simulink model "deployAGV_stateflow"  (R2024a)
settings: configuration reference "SharedConfig" (kept outside this file)
PostLoadFcn:
  | AGV_simulation
model workspace (MAT data in the model file):
  L = Simulink.Parameter
  L.Value = 2
  L.Complexity = 'real'
  L.Dimensions = [1 1]
  L.DataType = 'auto'
  mdlWSDbList = ["C:\Users\matlab.cut\Desktop\AMR\canbus_files\tramontina_database_xsens.dbc" "tramontina_database_curtis.dbc"]
  mdlWSDbcList = ["C:\Users\rodri\Dev\Projects\External\Tramontina\atlas\interface_models\xsens.dbc" "tramontina_database_curtis.dbc"]
  tfinal = Simulink.Parameter
  tfinal.Value = 350
  tfinal.Complexity = 'real'
  tfinal.Dimensions = [1 1]
  tfinal.DataType = 'auto'
undefined symbols (not defined in the file): DiscIntNeverNeededParam, magnitude, num_of_wps, T, T5, tstep
libraries: simulink x1, slrealtimeloglib x1
settings Model: DataDictionary=configuration_dictionary.sldd  Creator=rodri  LastModifiedBy=matlab.cut
settings ConfigSetRef: SourceName=SharedConfig

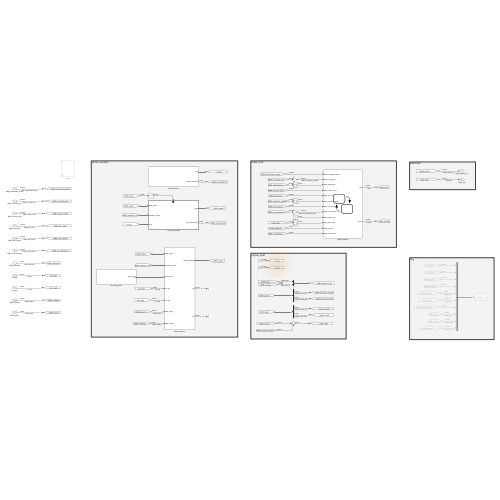
[thumbnail: Simulink's stored preview of the top-level diagram]
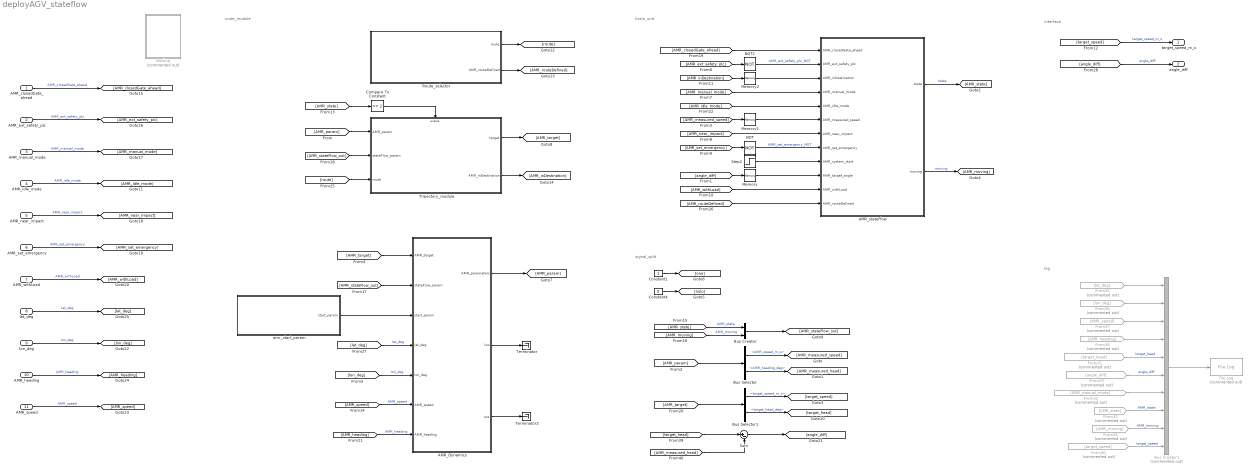
== system deployAGV_stateflow ==
  note: route_module
  note: brain_unit
  note: signal_split
  note: interface
  note: log
  AMR_closedGate_ahead : Inport  OutDataTypeStr=boolean
  AMR_ext_safety_plc : Inport  Port=2  OutDataTypeStr=boolean
  AMR_manual_mode : Inport  Port=3  OutDataTypeStr=boolean
  AMR_idle_mode : Inport  Port=4  OutDataTypeStr=boolean
  AMR_near_impact : Inport  Port=5  OutDataTypeStr=boolean
  AMR_set_emergency : Inport  Port=6  OutDataTypeStr=boolean
  AMR_withLoad : Inport  Port=7
  lat_deg : Inport  Port=8
  lon_deg : Inport  Port=9
  AMR_heading : Inport  Port=10
  AMR_speed : Inport  Port=11
  AMR_Dynamics : Subsystem
  AMR_stateFlow : Stateflow chart  TreatAsAtomicUnit=on
  Backup : Subsystem  Commented=on
  Bus Creator : BusCreator  Inputs=2
  Bus Creator1 : BusCreator  Commented=on  Inputs=10
  Bus Selector : BusSelector  OutputSignals=AMR_speed_m_s,AMR_heading_deg
  Bus Selector1 : BusSelector  OutputSignals=target_speed_m_s,target_head_deg
  Compare To Constant : simulink/Logic and Bit Operations/Compare To Constant  relop===  const=2  OutDataTypeStr=boolean
  Constant1 : Constant
  Constant4 : Constant  Value=0
  File Log : slrealtimeloglib/File Log  Commented=on  decimation=1  inputProcessing=Elements as channels (sample based)
  From29 : From  Commented=on  GotoTag=angle_diff
  From30 : From  Commented=on  GotoTag=target_speed
  From31 : From  Commented=on  GotoTag=target_head
  From32 : From  Commented=on  GotoTag=AMR_manual_mode
  From33 : From  Commented=on  GotoTag=AMR_state
  From34 : From  Commented=on  GotoTag=AMR_moving
  From35 : From  Commented=on  GotoTag=lat_deg
  From36 : From  Commented=on  GotoTag=lon_deg
  From37 : From  Commented=on  GotoTag=AMR_speed
  From38 : From  Commented=on  GotoTag=AMR_heading
  Memory : Memory
  Memory1 : Memory
  Memory2 : Memory
  NOT : Logic  Operator=NOT  IconShape=distinctive  AllPortsSameDT=off  OutDataTypeStr=boolean
  NOT1 : Logic  Operator=NOT  IconShape=distinctive  AllPortsSameDT=off  OutDataTypeStr=boolean
  Route_selector : Subsystem
  Step2 : Step  Time=10  SampleTime=0
  Sum : Sum  Inputs=|+-
  Terminator : Terminator
  Terminator2 : Terminator
  Trajectory_module : Subsystem
  amr_start_param : Subsystem
  target_speed_m_s : Outport
  angle_diff : Outport  Port=2
  wires:
  AMR_stateFlow/2(moving) -> [AMR_moving]  "moving"
  AMR_stateFlow/1(state) -> [AMR_state]  "state"
  [AMR_ext_safety_plc] -> NOT1/1
  [AMR_manual_mode] -> AMR_stateFlow/4(AMR_manual_mode)
  [AMR_measured_speed] -> Memory1/1
  [AMR_near_impact] -> AMR_stateFlow/7(AMR_near_impact)
  [AMR_set_emergency] -> NOT/1
  Step2/1 -> AMR_stateFlow/9(AMR_system_start)
  [angle_diff] -> Memory/1
  [AMR_withLoad] -> AMR_stateFlow/11(AMR_withLoad)
  [AMR_inDestination] -> Memory2/1
  [AMR_closedGate_ahead] -> AMR_stateFlow/1(AMR_closedGate_ahead)
  AMR_Dynamics/1(AMR_parameters) -> [AMR_param]
  [AMR_param] -> Trajectory_module/1(AMR_param)
  Trajectory_module/1(target) -> [AMR_target]
  [AMR_target] -> AMR_Dynamics/1(AMR_target)
  amr_start_param/1(start_param) -> AMR_Dynamics/3(start_param)
  [AMR_stateFlow_out] -> AMR_Dynamics/2(stateFlow_param)
  [AMR_stateFlow_out] -> Trajectory_module/2(stateFlow_param)
  [AMR_state] -> Compare To Constant/1
  Compare To Constant/1 -> Trajectory_module/Enable
  Memory/1 -> AMR_stateFlow/10(AMR_target_angle)
  Memory1/1 -> AMR_stateFlow/6(AMR_measured_speed)
  Route_selector/1(route) -> [route]
  Route_selector/2(AMR_routeDefined) -> [AMR_routeDefined]
  [route] -> Trajectory_module/3(route)
  [AMR_routeDefined] -> AMR_stateFlow/12(AMR_routeDefined)
  Trajectory_module/2(AMR_inDestination) -> [AMR_inDestination]
  Memory2/1 -> AMR_stateFlow/3(AMR_inDestination)
  AMR_closedGate_ahead/1 -> [AMR_closedGate_ahead]  "AMR_closedGate_ahead"
  AMR_manual_mode/1 -> [AMR_manual_mode]  "AMR_manual_mode"
  AMR_near_impact/1 -> [AMR_near_impact]  "AMR_near_impact"
  AMR_withLoad/1 -> [AMR_withLoad]  "AMR_withLoad"
  lat_deg/1 -> [lat_deg]  "lat_deg"
  [lat_deg] -> AMR_Dynamics/4(lat_deg)  "lat_deg"
  lon_deg/1 -> [lon_deg]  "lon_deg"
  AMR_speed/1 -> [AMR_speed]  "AMR_speed"
  AMR_heading/1 -> [AMR_heading]  "AMR_heading"
  [lon_deg] -> AMR_Dynamics/5(lon_deg)  "lon_deg"
  [AMR_speed] -> AMR_Dynamics/6(AMR_speed)  "AMR_speed"
  [AMR_heading] -> AMR_Dynamics/7(AMR_heading)  "AMR_heading"
  AMR_Dynamics/3(rws) -> Terminator2/1
  AMR_Dynamics/2(lws) -> Terminator/1
  AMR_set_emergency/1 -> [AMR_set_emergency]  "AMR_set_emergency"
  AMR_ext_safety_plc/1 -> [AMR_ext_safety_plc]  "AMR_ext_safety_plc"
  NOT1/1 -> AMR_stateFlow/2(AMR_ext_safety_plc)  "AMR_ext_safety_plc_NOT"
  NOT/1 -> AMR_stateFlow/8(AMR_set_emergency)  "AMR_set_emergency_NOT"
  Bus Creator/1 -> [AMR_stateFlow_out]
  [AMR_moving] -> Bus Creator/2  "AMR_moving"
  [AMR_state] -> Bus Creator/1  "AMR_state"
  Bus Selector/1 -> [AMR_measured_speed]  "<AMR_speed_m_s>"
  Bus Selector1/2 -> [target_head]  "<target_head_deg>"
  Constant1/1 -> [one]
  Constant4/1 -> [nulo]
  Bus Selector/2 -> [AMR_measured_head]  "<AMR_heading_deg>"
  Bus Selector1/1 -> [target_speed]  "<target_speed_m_s>"
  [AMR_param] -> Bus Selector/1
  [AMR_target] -> Bus Selector1/1
  [angle_diff] -> angle_diff/1  "angle_diff"
  [target_speed] -> target_speed_m_s/1  "target_speed_m_s"
  From38/1 -> Bus Creator1/4
  From31/1 -> Bus Creator1/5  "target_head"
  From35/1 -> Bus Creator1/1
  From36/1 -> Bus Creator1/2
  From29/1 -> Bus Creator1/6  "angle_diff"
  From34/1 -> Bus Creator1/9  "AMR_moving"
  From30/1 -> Bus Creator1/10  "target_speed"
  Bus Creator1/1 -> File Log/1
  From33/1 -> Bus Creator1/8  "AMR_state"
  From37/1 -> Bus Creator1/3
  From32/1 -> Bus Creator1/7
  [AMR_measured_head] -> Sum/2
  [target_head] -> Sum/1
  Sum/1 -> [angle_diff]
  AMR_idle_mode/1 -> [AMR_idle_mode]  "AMR_idle_mode"
  [AMR_idle_mode] -> AMR_stateFlow/5(AMR_idle_mode)

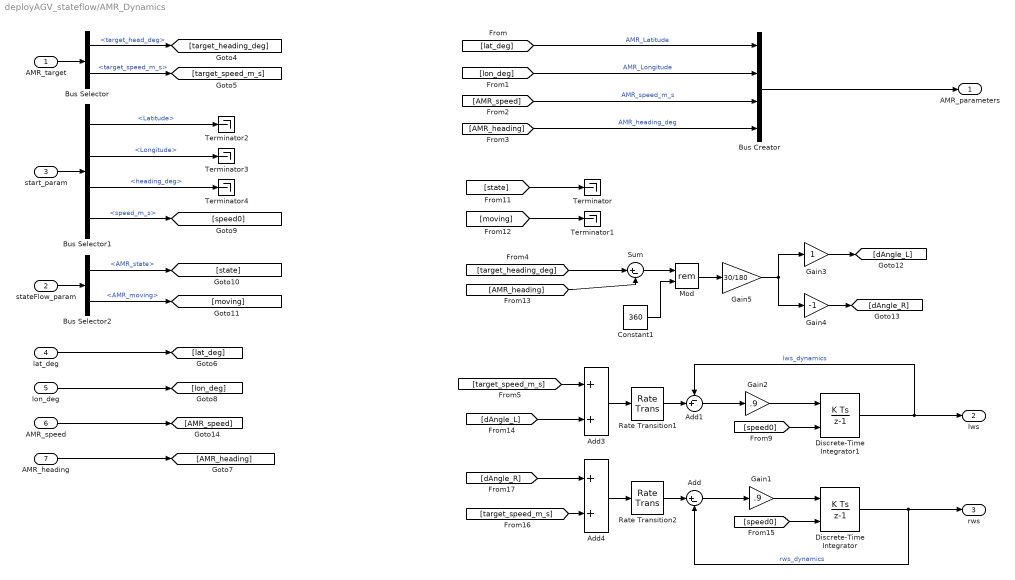
== system deployAGV_stateflow/AMR_Dynamics ==
  AMR_target : Inport
  stateFlow_param : Inport  Port=2
  start_param : Inport  Port=3
  lat_deg : Inport  Port=4
  lon_deg : Inport  Port=5
  AMR_speed : Inport  Port=6
  AMR_heading : Inport  Port=7
  Add : Sum  Inputs=|+-
  Add1 : Sum  Inputs=-+|
  Add3 : Sum
  Add4 : Sum
  Bus Creator : BusCreator  Inputs=4
  Bus Selector : BusSelector  OutputSignals=target_head_deg,target_speed_m_s
  Bus Selector1 : BusSelector  OutputSignals=Latitude,Longitude,heading_deg,speed_m_s
  Bus Selector2 : BusSelector  OutputSignals=AMR_state,AMR_moving
  Constant1 : Constant  Value=360
  Discrete-Time Integrator : DiscreteIntegrator  InitialConditionSource=external  SampleTime=tstep  ICPrevOutput=DiscIntNeverNeededParam  ICPrevScaledInput=DiscIntNeverNeededParam
  Discrete-Time Integrator1 : DiscreteIntegrator  InitialConditionSource=external  SampleTime=tstep  ICPrevOutput=DiscIntNeverNeededParam  ICPrevScaledInput=DiscIntNeverNeededParam
  Gain1 : Gain  Gain=.9
  Gain2 : Gain  Gain=.9
  Gain3 : Gain
  Gain4 : Gain  Gain=-1
  Gain5 : Gain  Gain=30/180
  Mod : Math  Operator=rem
  Rate Transition1 : RateTransition
  Rate Transition2 : RateTransition
  Sum : Sum  Inputs=|+-
  Terminator{,1..4} (5 alike) : Terminator
  AMR_parameters : Outport
  lws : Outport  Port=2
  rws : Outport  Port=3
  wires:
  [lat_deg] -> Bus Creator/1  "AMR_Latitude"
  [lon_deg] -> Bus Creator/2  "AMR_Longitude"
  Bus Creator/1 -> AMR_parameters/1
  [AMR_speed] -> Bus Creator/3  "AMR_speed_m_s"
  [AMR_heading] -> Bus Creator/4  "AMR_heading_deg"
  AMR_target/1 -> Bus Selector/1
  start_param/1 -> Bus Selector1/1
  Bus Selector/1 -> [target_heading_deg]  "<target_head_deg>"
  Bus Selector/2 -> [target_speed_m_s]  "<target_speed_m_s>"
  Bus Selector1/1 -> Terminator2/1  "<Latitude>"
  Bus Selector1/2 -> Terminator3/1  "<Longitude>"
  Bus Selector1/3 -> Terminator4/1  "<heading_deg>"
  Bus Selector1/4 -> [speed0]  "<speed_m_s>"
  [target_heading_deg] -> Sum/1
  stateFlow_param/1 -> Bus Selector2/1
  Bus Selector2/2 -> [moving]  "<AMR_moving>"
  Bus Selector2/1 -> [state]  "<AMR_state>"
  [state] -> Terminator/1
  [moving] -> Terminator1/1
  [AMR_heading] -> Sum/2
  Discrete-Time Integrator1/1 -> Add1/1, lws/1  "lws_dynamics"
  Discrete-Time Integrator/1 -> Add/2, rws/1  "rws_dynamics"
  [speed0] -> Discrete-Time Integrator/2
  Add/1 -> Gain1/1
  Add1/1 -> Gain2/1
  [speed0] -> Discrete-Time Integrator1/2
  Sum/1 -> Mod/1
  Constant1/1 -> Mod/2
  Gain3/1 -> [dAngle_L]
  Gain2/1 -> Discrete-Time Integrator1/1
  Gain1/1 -> Discrete-Time Integrator/1
  Gain4/1 -> [dAngle_R]
  Add3/1 -> Rate Transition1/1
  [target_speed_m_s] -> Add4/2
  Mod/1 -> Gain5/1
  [dAngle_R] -> Add4/1
  Gain5/1 -> Gain3/1, Gain4/1
  Add4/1 -> Rate Transition2/1
  lat_deg/1 -> [lat_deg]
  lon_deg/1 -> [lon_deg]
  AMR_speed/1 -> [AMR_speed]
  AMR_heading/1 -> [AMR_heading]
  [target_speed_m_s] -> Add3/1
  [dAngle_L] -> Add3/2
  Rate Transition1/1 -> Add1/2
  Rate Transition2/1 -> Add/1

== system deployAGV_stateflow/Backup ==
  Add : Sum  Inputs=+-
  Constant5 : Constant  Value=0
  GPS : Subsystem  Commented=on
  GPS_speed_measure : Subsystem  Commented=on
  Step : Step  Time=10  After=.000005  SampleTime=0
  Step1 : Step  Time=50  After=.000005  SampleTime=0
  wires:
  GPS_speed_measure/2(heading_deg) -> [agv_measured_heading]
  GPS/1(POS) -> [agv_pos]
  Constant5/1 -> GPS/1(dlat)
  Step1/1 -> Add/2
  Add/1 -> GPS/2(dlng)
  [agv_pos] -> GPS_speed_measure/1(GPS_POS)
  Step/1 -> Add/1
  GPS_speed_measure/1(speed_m_s) -> [agv_measured_speed]

== system deployAGV_stateflow/Route_selector ==
  Add : Sum  Inputs=+-
  Bus Creator4 : BusCreator  Inputs=2
  Constant : Constant
  Constant5 : Constant  Value=T.Latitude
  Constant9 : Constant  Value=T.Longitude
  Step : Step  Time=15  SampleTime=0
  Step1 : Step  Time=20  SampleTime=0
  Terminator : Terminator
  route : Outport
  AMR_routeDefined : Outport  Port=2
  wires:
  Bus Creator4/1 -> route/1  "route"
  Step/1 -> Add/1
  Step1/1 -> Add/2
  Constant9/1 -> Bus Creator4/2  "Longitude"
  Constant5/1 -> Bus Creator4/1  "Latitude"
  Constant/1 -> AMR_routeDefined/1
  Add/1 -> Terminator/1

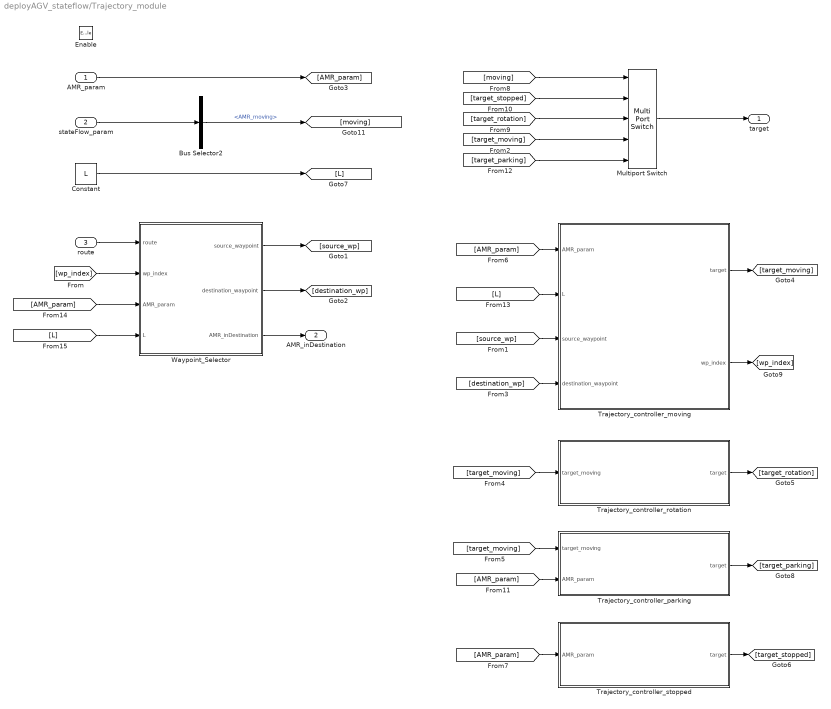
== system deployAGV_stateflow/Trajectory_module ==
  AMR_param : Inport
  stateFlow_param : Inport  Port=2
  route : Inport  Port=3
  Enable : EnablePort
  Bus Selector2 : BusSelector  OutputSignals=AMR_moving
  Constant : Constant  Value=L
  Multiport Switch : MultiPortSwitch  DataPortOrder=Zero-based contiguous  Inputs=4  zeroidx=on  SaturateOnIntegerOverflow=off  InputSameDT=off
  Trajectory_controller_moving : Subsystem
  Trajectory_controller_parking : Subsystem
  Trajectory_controller_rotation : Subsystem
  Trajectory_controller_stopped : Subsystem
  Waypoint_Selector : Subsystem
  target : Outport
  AMR_inDestination : Outport  Port=2
  wires:
  Trajectory_controller_moving/2(wp_index) -> [wp_index]
  [wp_index] -> Waypoint_Selector/2(wp_index)
  Trajectory_controller_moving/1(target) -> [target_moving]
  route/1 -> Waypoint_Selector/1(route)
  [L] -> Trajectory_controller_moving/2(L)
  Bus Selector2/1 -> [moving]  "<AMR_moving>"
  stateFlow_param/1 -> Bus Selector2/1
  [source_wp] -> Trajectory_controller_moving/3(source_waypoint)
  Waypoint_Selector/1(source_waypoint) -> [source_wp]
  Waypoint_Selector/2(destination_waypoint) -> [destination_wp]
  [destination_wp] -> Trajectory_controller_moving/4(destination_waypoint)
  AMR_param/1 -> [AMR_param]
  [AMR_param] -> Trajectory_controller_moving/1(AMR_param)
  Trajectory_controller_rotation/1(target) -> [target_rotation]
  Multiport Switch/1 -> target/1
  [moving] -> Multiport Switch/1
  [target_stopped] -> Multiport Switch/2
  [target_parking] -> Multiport Switch/5
  [target_moving] -> Multiport Switch/4
  [target_rotation] -> Multiport Switch/3
  [target_moving] -> Trajectory_controller_rotation/1(target_moving)
  [target_moving] -> Trajectory_controller_parking/1(target_moving)
  Trajectory_controller_parking/1(target) -> [target_parking]
  [AMR_param] -> Trajectory_controller_parking/2(AMR_param)
  [AMR_param] -> Trajectory_controller_stopped/1(AMR_param)
  Trajectory_controller_stopped/1(target) -> [target_stopped]
  Constant/1 -> [L]
  [AMR_param] -> Waypoint_Selector/3(AMR_param)
  [L] -> Waypoint_Selector/4(L)
  Waypoint_Selector/3(AMR_inDestination) -> AMR_inDestination/1

== system deployAGV_stateflow/amr_start_param ==
  Bus Creator : BusCreator  Inputs=4
  Constant : Constant  Value=T5.Latitude(1)
  Constant1 : Constant  Value=T5.Longitude(1)
  Constant2 : Constant  Value=0
  Constant3 : Constant  Value=0
  start_param : Outport
  wires:
  Bus Creator/1 -> start_param/1
  Constant/1 -> Bus Creator/1  "Latitude"
  Constant1/1 -> Bus Creator/2  "Longitude"
  Constant2/1 -> Bus Creator/3  "heading_deg"
  Constant3/1 -> Bus Creator/4  "speed_m_s"

== system deployAGV_stateflow/Backup/GPS ==
  dlat : Inport
  dlng : Inport  Port=2
  Add : Sum  Inputs=|++
  Add1 : Sum  Inputs=|++
  Matrix Concatenate : Concatenate  Mode=Multidimensional array  ConcatenateDimension=2
  lat : Memory  InitialCondition=-29.272334
  lng : Memory  InitialCondition=-51.467679
  POS : Outport
  wires:
  lat/1 -> Add1/2, Matrix Concatenate/1
  Matrix Concatenate/1 -> POS/1
  dlat/1 -> Add1/1
  Add1/1 -> lat/1
  lng/1 -> Add/2, Matrix Concatenate/2
  Add/1 -> lng/1
  dlng/1 -> Add/1

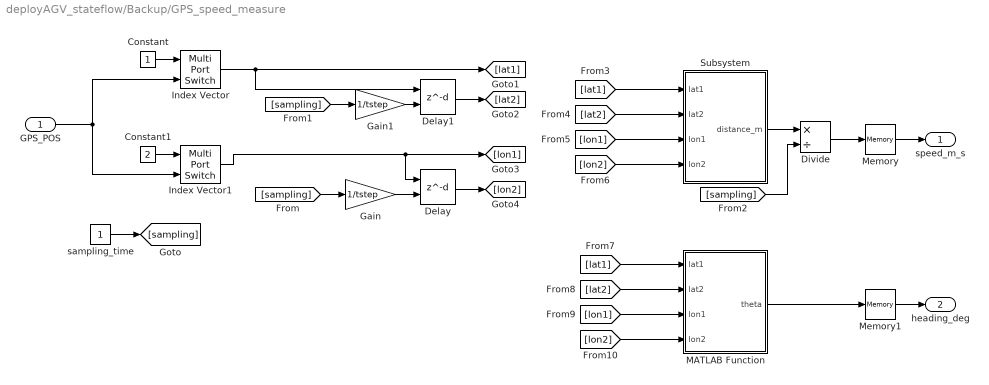
== system deployAGV_stateflow/Backup/GPS_speed_measure ==
  GPS_POS : Inport
  Constant : Constant
  Constant1 : Constant  Value=2
  Delay : Delay  DelayLengthSource=Input port  DelayLength=5/tstep  InitialCondition=-51.467679
      settings: InputPortMap=u0,p1
  Delay1 : Delay  DelayLengthSource=Input port  DelayLength=5/tstep  InitialCondition=-29.272334
      settings: InputPortMap=u0,p1
  Divide : Product  Inputs=*/
  Gain : Gain  Gain=1/tstep
  Gain1 : Gain  Gain=1/tstep
  Index Vector : MultiPortSwitch  Inputs=1  SaturateOnIntegerOverflow=off  InputSameDT=off
  Index Vector1 : MultiPortSwitch  Inputs=1  SaturateOnIntegerOverflow=off  InputSameDT=off
  MATLAB Function : MATLAB Function  TreatAsAtomicUnit=on
  Memory : Memory
  Memory1 : Memory
  Subsystem : Subsystem
  sampling_time : Constant
  speed_m_s : Outport
  heading_deg : Outport  Port=2
  wires:
  Subsystem/1(distance_m) -> Divide/1
  Memory/1 -> speed_m_s/1
  Divide/1 -> Memory/1
  Constant/1 -> Index Vector/1
  Constant1/1 -> Index Vector1/1
  Index Vector1/1 -> [lon1], Delay/1
  sampling_time/1 -> [sampling]
  Gain/1 -> Delay/2
  [sampling] -> Gain/1
  [sampling] -> Gain1/1
  Gain1/1 -> Delay1/2
  Index Vector/1 -> [lat1], Delay1/1
  GPS_POS/1 -> Index Vector/2, Index Vector1/2
  [sampling] -> Divide/2
  Memory1/1 -> heading_deg/1
  Delay1/1 -> [lat2]
  Delay/1 -> [lon2]
  [lat2] -> Subsystem/2(lat2)
  [lon1] -> Subsystem/3(lon1)
  [lon2] -> Subsystem/4(lon2)
  [lat1] -> Subsystem/1(lat1)
  [lon2] -> MATLAB Function/4(lon2)
  [lat1] -> MATLAB Function/1(lat1)
  [lon1] -> MATLAB Function/3(lon1)
  [lat2] -> MATLAB Function/2(lat2)
  MATLAB Function/1(theta) -> Memory1/1

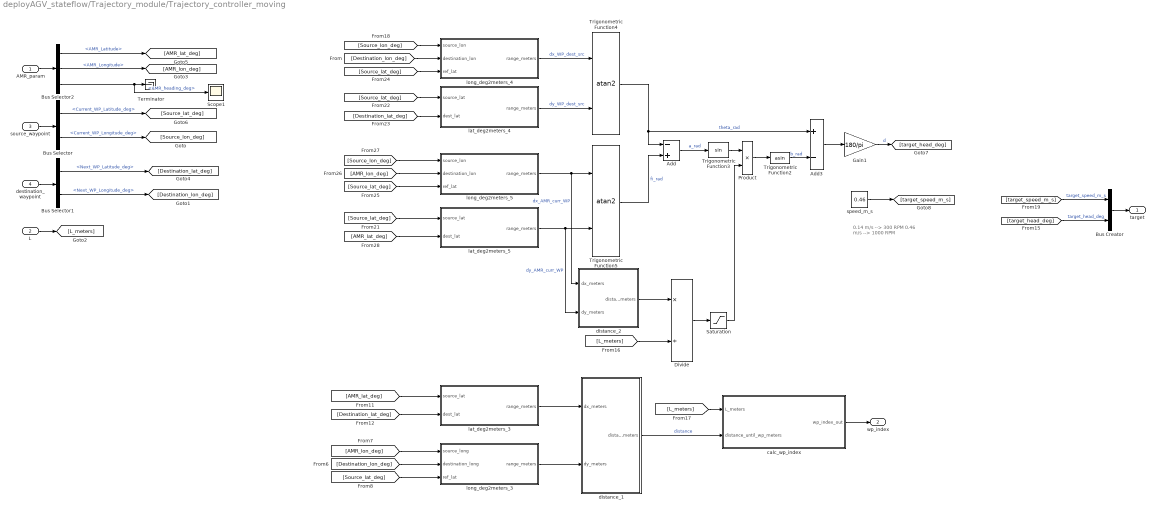
== system deployAGV_stateflow/Trajectory_module/Trajectory_controller_moving ==
  note: 0.14 m/s --> 300 RPM
      | 0.46 m/s --> 1000 RPM
  AMR_param : Inport
  L : Inport  Port=2
  source_waypoint : Inport  Port=3
  destination_waypoint : Inport  Port=4
  Add : Sum  Inputs=-+
  Add3 : Sum  Inputs=+-
  Bus Creator : BusCreator  Inputs=2
  Bus Selector : BusSelector  OutputSignals=Current_WP_Latitude_deg,Current_WP_Longitude_deg
  Bus Selector1 : BusSelector  OutputSignals=Next_WP_Latitude_deg,Next_WP_Longitude_deg
  Bus Selector2 : BusSelector  OutputSignals=AMR_Latitude,AMR_Longitude,AMR_heading_deg
  Divide : Product  Inputs=*/
  Gain1 : Gain  Gain=180/pi
  Product : Product
  Saturation : Saturate  UpperLimit=1  LowerLimit=0
  Scope1 : Scope
  Terminator : Terminator
  Trigonometric Function2 : Trigonometry  Operator=asin
  Trigonometric Function3 : Trigonometry
  Trigonometric Function4 : Trigonometry  Operator=atan2
  Trigonometric Function5 : Trigonometry  Operator=atan2
  calc_wp_index : Subsystem
  distance_1 : Subsystem  TreatAsAtomicUnit=on
  distance_2 : Subsystem  TreatAsAtomicUnit=on
  lat_deg2meters_3 : Subsystem  TreatAsAtomicUnit=on
  lat_deg2meters_4 : Subsystem  TreatAsAtomicUnit=on
  lat_deg2meters_5 : Subsystem  TreatAsAtomicUnit=on
  long_deg2meters_3 : Subsystem  TreatAsAtomicUnit=on
  long_deg2meters_4 : Subsystem  TreatAsAtomicUnit=on
  long_deg2meters_5 : Subsystem  TreatAsAtomicUnit=on
  speed_m_s : Constant  Value=0.46
  target : Outport
  wp_index : Outport  Port=2
  wires:
  distance_1/1(distance_meters) -> calc_wp_index/2(distance_until_wp_meters)  "distance"
  calc_wp_index/1(wp_index_out) -> wp_index/1
  [Destination_lon_deg] -> long_deg2meters_3/2(destination_long)
  [Source_lat_deg] -> long_deg2meters_3/3(ref_lat)
  Trigonometric Function4/1 -> Add3/1, Add/1  "theta_rad"
  [L_meters] -> Divide/2
  [L_meters] -> calc_wp_index/1(L_meters)
  source_waypoint/1 -> Bus Selector/1
  destination_waypoint/1 -> Bus Selector1/1
  AMR_param/1 -> Bus Selector2/1
  Bus Selector2/1 -> [AMR_lat_deg]  "<AMR_Latitude>"
  Bus Selector2/2 -> [AMR_lon_deg]  "<AMR_Longitude>"
  Bus Selector/1 -> [Source_lat_deg]  "<Current_WP_Latitude_deg>"
  Bus Selector1/2 -> [Destination_lon_deg]  "<Next_WP_Longitude_deg>"
  Bus Selector1/1 -> [Destination_lat_deg]  "<Next_WP_Latitude_deg>"
  Bus Selector/2 -> [Source_lon_deg]  "<Current_WP_Longitude_deg>"
  [AMR_lon_deg] -> long_deg2meters_3/1(source_long)
  L/1 -> [L_meters]
  [target_speed_m_s] -> Bus Creator/1  "target_speed_m_s"
  [target_head_deg] -> Bus Creator/2  "target_head_deg"
  Bus Creator/1 -> target/1
  Add/1 -> Trigonometric Function3/1  "a_rad"
  Trigonometric Function3/1 -> Product/1
  speed_m_s/1 -> [target_speed_m_s]
  Bus Selector2/3 -> Scope1/1, Terminator/1  "<AMR_heading_deg>"
  Gain1/1 -> [target_head_deg]  "d"
  distance_2/1(distance_meters) -> Divide/1
  [Destination_lat_deg] -> lat_deg2meters_3/2(dest_lat)
  [AMR_lat_deg] -> lat_deg2meters_3/1(source_lat)
  Trigonometric Function5/1 -> Add/2  "fi_rad"
  lat_deg2meters_3/1(range_meters) -> distance_1/1(dx_meters)
  long_deg2meters_3/1(range_meters) -> distance_1/2(dy_meters)
  long_deg2meters_4/1(range_meters) -> Trigonometric Function4/1  "dx_WP_dest_src"
  lat_deg2meters_4/1(range_meters) -> Trigonometric Function4/2  "dy_WP_dest_src"
  long_deg2meters_5/1(range_meters) -> distance_2/1(dx_meters), Trigonometric Function5/1  "dx_AMR_curr_WP"
  lat_deg2meters_5/1(range_meters) -> distance_2/2(dy_meters), Trigonometric Function5/2  "dy_AMR_curr_WP"
  Add3/1 -> Gain1/1
  [Source_lon_deg] -> long_deg2meters_5/1(source_lon)
  [Source_lat_deg] -> long_deg2meters_4/3(ref_lat)
  [Source_lat_deg] -> lat_deg2meters_4/1(source_lat)
  [Destination_lon_deg] -> long_deg2meters_4/2(destination_lon)
  [AMR_lon_deg] -> long_deg2meters_5/2(destination_lon)
  [Source_lat_deg] -> long_deg2meters_5/3(ref_lat)
  [Destination_lat_deg] -> lat_deg2meters_4/2(dest_lat)
  [Source_lat_deg] -> lat_deg2meters_5/1(source_lat)
  [Source_lon_deg] -> long_deg2meters_4/1(source_lon)
  [AMR_lat_deg] -> lat_deg2meters_5/2(dest_lat)
  Trigonometric Function2/1 -> Add3/2  "b_rad"
  Product/1 -> Trigonometric Function2/1
  Divide/1 -> Saturation/1
  Saturation/1 -> Product/2

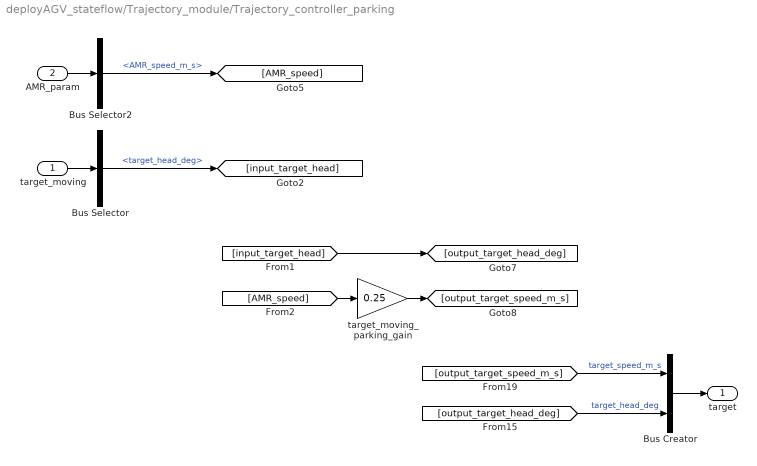
== system deployAGV_stateflow/Trajectory_module/Trajectory_controller_parking ==
  target_moving : Inport
  AMR_param : Inport  Port=2
  Bus Creator : BusCreator  Inputs=2
  Bus Selector : BusSelector  OutputSignals=target_head_deg
  Bus Selector2 : BusSelector  OutputSignals=AMR_speed_m_s
  target_moving_parking_gain : Gain  Gain=0.25
  target : Outport
  wires:
  [output_target_speed_m_s] -> Bus Creator/1  "target_speed_m_s"
  [output_target_head_deg] -> Bus Creator/2  "target_head_deg"
  Bus Creator/1 -> target/1
  [input_target_head] -> [output_target_head_deg]
  target_moving/1 -> Bus Selector/1
  AMR_param/1 -> Bus Selector2/1
  Bus Selector2/1 -> [AMR_speed]  "<AMR_speed_m_s>"
  Bus Selector/1 -> [input_target_head]  "<target_head_deg>"
  target_moving_parking_gain/1 -> [output_target_speed_m_s]
  [AMR_speed] -> target_moving_parking_gain/1

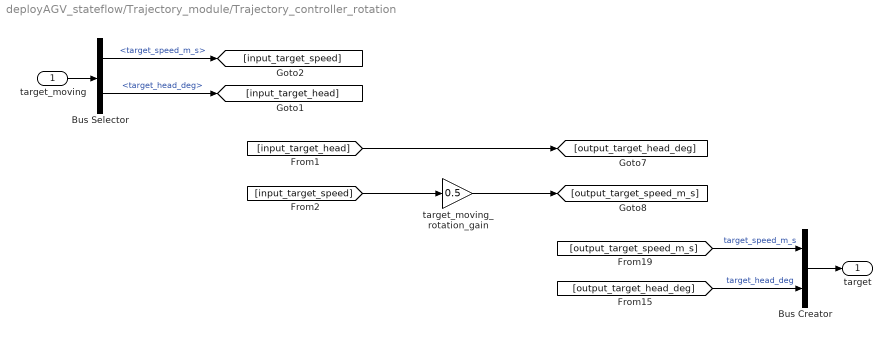
== system deployAGV_stateflow/Trajectory_module/Trajectory_controller_rotation ==
  target_moving : Inport
  Bus Creator : BusCreator  Inputs=2
  Bus Selector : BusSelector  OutputSignals=target_speed_m_s,target_head_deg
  target_moving_rotation_gain : Gain  Gain=0.5
  target : Outport
  wires:
  [output_target_speed_m_s] -> Bus Creator/1  "target_speed_m_s"
  [output_target_head_deg] -> Bus Creator/2  "target_head_deg"
  Bus Creator/1 -> target/1
  target_moving/1 -> Bus Selector/1
  Bus Selector/1 -> [input_target_speed]  "<target_speed_m_s>"
  Bus Selector/2 -> [input_target_head]  "<target_head_deg>"
  [input_target_speed] -> target_moving_rotation_gain/1
  [input_target_head] -> [output_target_head_deg]
  target_moving_rotation_gain/1 -> [output_target_speed_m_s]

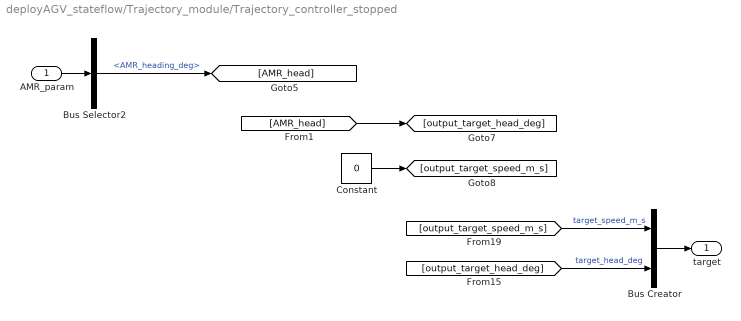
== system deployAGV_stateflow/Trajectory_module/Trajectory_controller_stopped ==
  AMR_param : Inport
  Bus Creator : BusCreator  Inputs=2
  Bus Selector2 : BusSelector  OutputSignals=AMR_heading_deg
  Constant : Constant  Value=0
  target : Outport
  wires:
  [output_target_speed_m_s] -> Bus Creator/1  "target_speed_m_s"
  [output_target_head_deg] -> Bus Creator/2  "target_head_deg"
  Bus Creator/1 -> target/1
  [AMR_head] -> [output_target_head_deg]
  AMR_param/1 -> Bus Selector2/1
  Bus Selector2/1 -> [AMR_head]  "<AMR_heading_deg>"
  Constant/1 -> [output_target_speed_m_s]

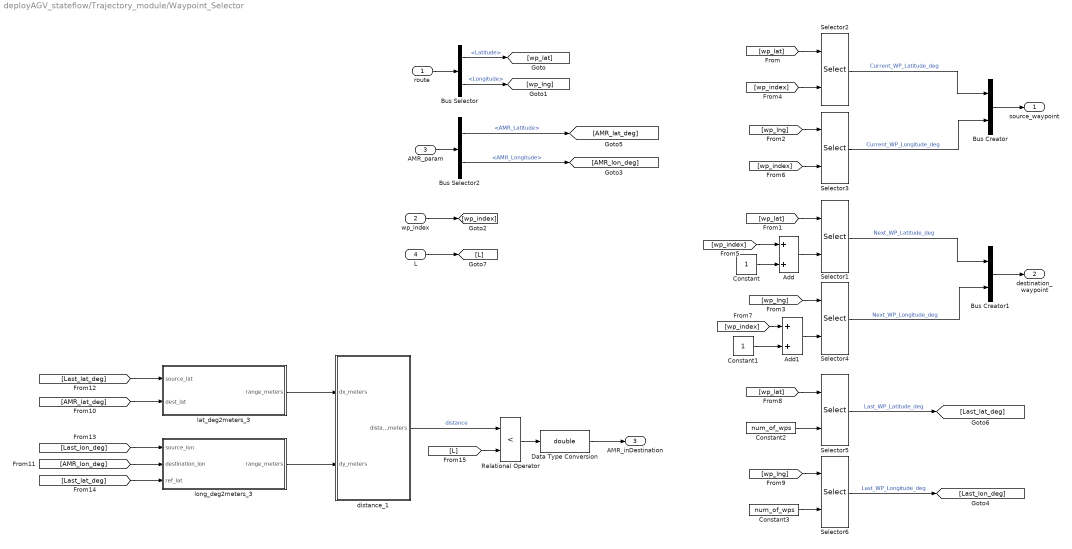
== system deployAGV_stateflow/Trajectory_module/Waypoint_Selector ==
  route : Inport
  wp_index : Inport  Port=2
  AMR_param : Inport  Port=3
  L : Inport  Port=4
  Add : Sum
  Add1 : Sum
  Bus Creator : BusCreator  Inputs=2
  Bus Creator1 : BusCreator  Inputs=2
  Bus Selector : BusSelector  OutputSignals=Latitude,Longitude
  Bus Selector2 : BusSelector  OutputSignals=AMR_Latitude,AMR_Longitude
  Constant : Constant
  Constant1 : Constant
  Constant2 : Constant  Value=num_of_wps
  Constant3 : Constant  Value=num_of_wps
  Data Type Conversion : DataTypeConversion  OutDataTypeStr=double  SaturateOnIntegerOverflow=off  RndMeth=Floor
  Relational Operator : RelationalOperator  Operator=<  OutDataTypeStr=boolean  RndMeth=Simplest  InputSameDT=off
  Selector{1..6} (6 alike) : Selector  InputPortWidth=num_of_wps  IndexOptions=Index vector (port)  Indices=[1 3]  OutputSizes=1
  distance_1 : Subsystem  TreatAsAtomicUnit=on
  lat_deg2meters_3 : Subsystem  TreatAsAtomicUnit=on
  long_deg2meters_3 : Subsystem  TreatAsAtomicUnit=on
  source_waypoint : Outport
  destination_waypoint : Outport  Port=2
  AMR_inDestination : Outport  Port=3
  wires:
  Selector2/1 -> Bus Creator/1  "Current_WP_Latitude_deg"
  Add/1 -> Selector1/2
  Constant/1 -> Add/2
  Constant1/1 -> Add1/2
  Add1/1 -> Selector4/2
  route/1 -> Bus Selector/1
  Bus Selector/1 -> [wp_lat]  "<Latitude>"
  Bus Selector/2 -> [wp_lng]  "<Longitude>"
  [wp_lat] -> Selector2/1
  [wp_lat] -> Selector1/1
  [wp_lng] -> Selector3/1
  [wp_lng] -> Selector4/1
  wp_index/1 -> [wp_index]
  [wp_index] -> Selector2/2
  [wp_index] -> Add/1
  [wp_index] -> Selector3/2
  [wp_index] -> Add1/1
  Bus Creator/1 -> source_waypoint/1
  Selector3/1 -> Bus Creator/2  "Current_WP_Longitude_deg"
  Selector4/1 -> Bus Creator1/2  "Next_WP_Longitude_deg"
  Selector1/1 -> Bus Creator1/1  "Next_WP_Latitude_deg"
  Bus Creator1/1 -> destination_waypoint/1
  Bus Selector2/1 -> [AMR_lat_deg]  "<AMR_Latitude>"
  AMR_param/1 -> Bus Selector2/1
  Bus Selector2/2 -> [AMR_lon_deg]  "<AMR_Longitude>"
  [wp_lat] -> Selector5/1
  [wp_lng] -> Selector6/1
  Constant3/1 -> Selector6/2
  Constant2/1 -> Selector5/2
  long_deg2meters_3/1(range_meters) -> distance_1/2(dy_meters)
  lat_deg2meters_3/1(range_meters) -> distance_1/1(dx_meters)
  Selector5/1 -> [Last_lat_deg]  "Last_WP_Latitude_deg"
  Selector6/1 -> [Last_lon_deg]  "Last_WP_Longitude_deg"
  [Last_lat_deg] -> lat_deg2meters_3/1(source_lat)
  [Last_lon_deg] -> long_deg2meters_3/1(source_lon)
  [Last_lat_deg] -> long_deg2meters_3/3(ref_lat)
  [AMR_lat_deg] -> lat_deg2meters_3/2(dest_lat)
  [AMR_lon_deg] -> long_deg2meters_3/2(destination_lon)
  Relational Operator/1 -> Data Type Conversion/1
  distance_1/1(distance_meters) -> Relational Operator/1  "distance"
  L/1 -> [L]
  [L] -> Relational Operator/2
  Data Type Conversion/1 -> AMR_inDestination/1

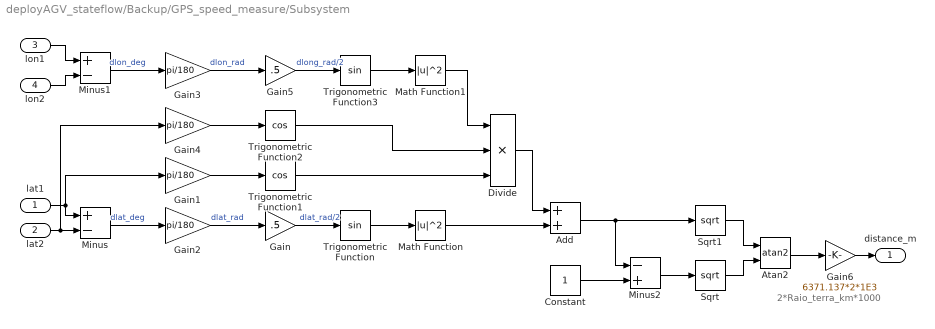
== system deployAGV_stateflow/Backup/GPS_speed_measure/Subsystem ==
  note: 2*Raio_terra_km*1000
  lat1 : Inport
  lat2 : Inport  Port=2
  lon1 : Inport  Port=3
  lon2 : Inport  Port=4
  Add : Sum
  Atan2 : Trigonometry  Operator=atan2
  Constant : Constant
  Divide : Product  Inputs=***
  Gain : Gain  Gain=.5
  Gain{1..4} (4 alike) : Gain  Gain=pi/180
  Gain5 : Gain  Gain=.5
  Gain6 : Gain  Gain=6371.137*2*1E3
  Math Function : Math  Operator=magnitude^2
  Math Function1 : Math  Operator=magnitude^2
  Minus : Sum  Inputs=+-
  Minus1 : Sum  Inputs=+-
  Minus2 : Sum  Inputs=-+
  Sqrt : Sqrt
  Sqrt1 : Sqrt
  Trigonometric Function : Trigonometry
  Trigonometric Function1 : Trigonometry  Operator=cos
  Trigonometric Function2 : Trigonometry  Operator=cos
  Trigonometric Function3 : Trigonometry
  distance_m : Outport
  wires:
  Minus/1 -> Gain2/1  "dlat_deg"
  Minus1/1 -> Gain3/1  "dlon_deg"
  lat2/1 -> Gain4/1, Minus/2
  lat1/1 -> Gain1/1, Minus/1
  lon1/1 -> Minus1/1
  lon2/1 -> Minus1/2
  Gain2/1 -> Gain/1  "dlat_rad"
  Gain/1 -> Trigonometric Function/1  "dlat_rad/2"
  Trigonometric Function/1 -> Math Function/1
  Math Function/1 -> Add/2
  Gain1/1 -> Trigonometric Function1/1
  Gain4/1 -> Trigonometric Function2/1
  Divide/1 -> Add/1
  Trigonometric Function3/1 -> Math Function1/1
  Gain5/1 -> Trigonometric Function3/1  "dlong_rad/2"
  Gain3/1 -> Gain5/1  "dlon_rad"
  Trigonometric Function1/1 -> Divide/3
  Trigonometric Function2/1 -> Divide/2
  Math Function1/1 -> Divide/1
  Add/1 -> Minus2/1, Sqrt1/1
  Minus2/1 -> Sqrt/1
  Atan2/1 -> Gain6/1
  Gain6/1 -> distance_m/1
  Constant/1 -> Minus2/2
  Sqrt1/1 -> Atan2/1
  Sqrt/1 -> Atan2/2

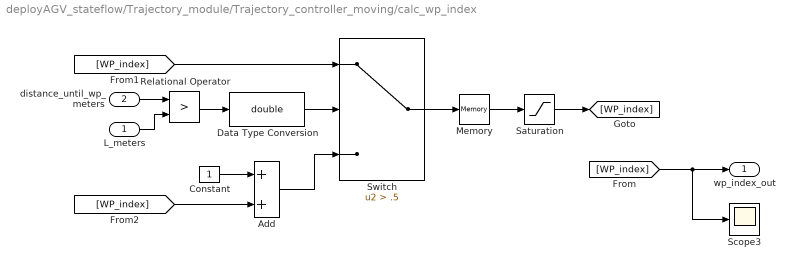
== system deployAGV_stateflow/Trajectory_module/Trajectory_controller_moving/calc_wp_index ==
  L_meters : Inport
  distance_until_wp_meters : Inport  Port=2
  Add : Sum
  Constant : Constant
  Data Type Conversion : DataTypeConversion  OutDataTypeStr=double  SaturateOnIntegerOverflow=off  RndMeth=Floor
  Memory : Memory  InitialCondition=1
  Relational Operator : RelationalOperator  Operator=>  OutDataTypeStr=boolean  RndMeth=Simplest  InputSameDT=off
  Saturation : Saturate  UpperLimit=num_of_wps-1  LowerLimit=1
  Scope3 : Scope
  Switch : Switch  Criteria=u2 > Threshold  Threshold=.5  SaturateOnIntegerOverflow=off  InputSameDT=off
  wp_index_out : Outport
  wires:
  distance_until_wp_meters/1 -> Relational Operator/1
  L_meters/1 -> Relational Operator/2
  Relational Operator/1 -> Data Type Conversion/1
  Data Type Conversion/1 -> Switch/2
  Switch/1 -> Memory/1
  Add/1 -> Switch/3
  Constant/1 -> Add/1
  [WP_index] -> wp_index_out/1, Scope3/1
  [WP_index] -> Switch/1
  [WP_index] -> Add/2
  Saturation/1 -> [WP_index]
  Memory/1 -> Saturation/1

== system deployAGV_stateflow/Trajectory_module/Trajectory_controller_moving/distance_1 ==
  dx_meters : Inport
  dy_meters : Inport  Port=2
  Add : Sum
  Divide1 : Product  Inputs=**
  Divide2 : Product  Inputs=**
  Sqrt : Sqrt
  distance_meters : Outport
  wires:
  dx_meters/1 -> Divide1/2, Divide1/1
  Divide1/1 -> Add/1
  Add/1 -> Sqrt/1
  dy_meters/1 -> Divide2/2, Divide2/1
  Divide2/1 -> Add/2
  Sqrt/1 -> distance_meters/1

== system deployAGV_stateflow/Trajectory_module/Trajectory_controller_moving/distance_2 ==
  dx_meters : Inport
  dy_meters : Inport  Port=2
  Add : Sum
  Divide1 : Product  Inputs=**
  Divide2 : Product  Inputs=**
  Sqrt : Sqrt
  distance_meters : Outport
  wires:
  dx_meters/1 -> Divide1/2, Divide1/1
  Divide1/1 -> Add/1
  Add/1 -> Sqrt/1
  dy_meters/1 -> Divide2/2, Divide2/1
  Divide2/1 -> Add/2
  Sqrt/1 -> distance_meters/1

== system deployAGV_stateflow/Trajectory_module/Trajectory_controller_moving/lat_deg2meters_3 ==
  source_lat : Inport
  dest_lat : Inport  Port=2
  Add : Sum  Inputs=+-
  deg2meters : Gain  Gain=111195
  range_meters : Outport
  wires:
  Add/1 -> deg2meters/1
  deg2meters/1 -> range_meters/1
  dest_lat/1 -> Add/1
  source_lat/1 -> Add/2

== system deployAGV_stateflow/Trajectory_module/Trajectory_controller_moving/lat_deg2meters_4 ==
  source_lat : Inport
  dest_lat : Inport  Port=2
  Add : Sum  Inputs=+-
  deg2meters : Gain  Gain=111195
  range_meters : Outport
  wires:
  Add/1 -> deg2meters/1
  deg2meters/1 -> range_meters/1
  dest_lat/1 -> Add/1
  source_lat/1 -> Add/2

== system deployAGV_stateflow/Trajectory_module/Trajectory_controller_moving/lat_deg2meters_5 ==
  source_lat : Inport
  dest_lat : Inport  Port=2
  Add : Sum  Inputs=+-
  deg2meters : Gain  Gain=111195
  range_meters : Outport
  wires:
  Add/1 -> deg2meters/1
  deg2meters/1 -> range_meters/1
  dest_lat/1 -> Add/1
  source_lat/1 -> Add/2

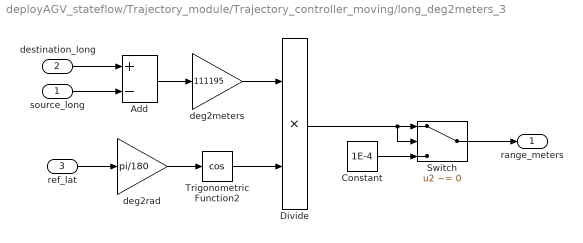
== system deployAGV_stateflow/Trajectory_module/Trajectory_controller_moving/long_deg2meters_3 ==
  source_long : Inport
  destination_long : Inport  Port=2
  ref_lat : Inport  Port=3
  Add : Sum  Inputs=+-
  Constant : Constant  Value=1E-4
  Divide : Product  Inputs=**
  Switch : Switch  Criteria=u2 ~= 0  SaturateOnIntegerOverflow=off  InputSameDT=off
  Trigonometric Function2 : Trigonometry  Operator=cos
  deg2meters : Gain  Gain=111195
  deg2rad : Gain  Gain=pi/180
  range_meters : Outport
  wires:
  Trigonometric Function2/1 -> Divide/2
  deg2rad/1 -> Trigonometric Function2/1
  ref_lat/1 -> deg2rad/1
  Constant/1 -> Switch/3
  source_long/1 -> Add/2
  Add/1 -> deg2meters/1
  deg2meters/1 -> Divide/1
  Switch/1 -> range_meters/1
  destination_long/1 -> Add/1
  Divide/1 -> Switch/2, Switch/1

== system deployAGV_stateflow/Trajectory_module/Trajectory_controller_moving/long_deg2meters_4 ==
  source_lon : Inport
  destination_lon : Inport  Port=2
  ref_lat : Inport  Port=3
  Add : Sum  Inputs=+-
  Divide : Product  Inputs=**
  Trigonometric Function2 : Trigonometry  Operator=cos
  deg2meters : Gain  Gain=111195
  deg2rad : Gain  Gain=pi/180
  range_meters : Outport
  wires:
  Trigonometric Function2/1 -> Divide/2
  deg2rad/1 -> Trigonometric Function2/1
  ref_lat/1 -> deg2rad/1
  source_lon/1 -> Add/2
  Add/1 -> deg2meters/1
  deg2meters/1 -> Divide/1
  Divide/1 -> range_meters/1
  destination_lon/1 -> Add/1

== system deployAGV_stateflow/Trajectory_module/Trajectory_controller_moving/long_deg2meters_5 ==
  source_lon : Inport
  destination_lon : Inport  Port=2
  ref_lat : Inport  Port=3
  Add : Sum  Inputs=+-
  Divide : Product  Inputs=**
  Trigonometric Function2 : Trigonometry  Operator=cos
  deg2meters : Gain  Gain=111195
  deg2rad : Gain  Gain=pi/180
  range_meters : Outport
  wires:
  Trigonometric Function2/1 -> Divide/2
  deg2rad/1 -> Trigonometric Function2/1
  ref_lat/1 -> deg2rad/1
  source_lon/1 -> Add/2
  Add/1 -> deg2meters/1
  deg2meters/1 -> Divide/1
  destination_lon/1 -> Add/1
  Divide/1 -> range_meters/1

== system deployAGV_stateflow/Trajectory_module/Waypoint_Selector/distance_1 ==
  dx_meters : Inport
  dy_meters : Inport  Port=2
  Add : Sum
  Divide1 : Product  Inputs=**
  Divide2 : Product  Inputs=**
  Sqrt : Sqrt
  distance_meters : Outport
  wires:
  dx_meters/1 -> Divide1/2, Divide1/1
  Divide1/1 -> Add/1
  Add/1 -> Sqrt/1
  dy_meters/1 -> Divide2/2, Divide2/1
  Divide2/1 -> Add/2
  Sqrt/1 -> distance_meters/1

== system deployAGV_stateflow/Trajectory_module/Waypoint_Selector/lat_deg2meters_3 ==
  source_lat : Inport
  dest_lat : Inport  Port=2
  Add : Sum  Inputs=+-
  deg2meters : Gain  Gain=111195
  range_meters : Outport
  wires:
  Add/1 -> deg2meters/1
  deg2meters/1 -> range_meters/1
  dest_lat/1 -> Add/1
  source_lat/1 -> Add/2

== system deployAGV_stateflow/Trajectory_module/Waypoint_Selector/long_deg2meters_3 ==
  source_lon : Inport
  destination_lon : Inport  Port=2
  ref_lat : Inport  Port=3
  Add : Sum  Inputs=+-
  Constant : Constant  Value=1E-4
  Divide : Product  Inputs=**
  Switch : Switch  Criteria=u2 ~= 0  SaturateOnIntegerOverflow=off  InputSameDT=off
  Trigonometric Function2 : Trigonometry  Operator=cos
  deg2meters : Gain  Gain=111195
  deg2rad : Gain  Gain=pi/180
  range_meters : Outport
  wires:
  Trigonometric Function2/1 -> Divide/2
  deg2rad/1 -> Trigonometric Function2/1
  ref_lat/1 -> deg2rad/1
  Constant/1 -> Switch/3
  source_lon/1 -> Add/2
  Add/1 -> deg2meters/1
  deg2meters/1 -> Divide/1
  Switch/1 -> range_meters/1
  destination_lon/1 -> Add/1
  Divide/1 -> Switch/2, Switch/1

== matlab function deployAGV_stateflow/Backup/GPS_speed_measure/MATLAB Function ==
  data: lat1 input; theta output; lat2 input; lon1 input; lon2 input
function theta = angle(lat1, lat2, lon1, lon2)
    lat2 = lat2 * pi/180;
    lat1 = lat1 * pi/180;
    lon1 = lon1 * pi/180;
    lon2 = lon2 * pi/180;
    
    t1 = tan( lat2/2 + pi/4 );
    t2 = tan( lat1/2 + pi/4);
    dphi = log(t1/t2);
    dlon = abs(lon1-lon2);
    theta = atan2( mod(dlon, 180) , dphi)*180/pi;

== stateflow chart deployAGV_stateflow/AMR_stateFlow ==
  note: Constantes:
      | WAITING = 0
      | SUCCESS=1
      | FAIL=-1
      | FALSE=0
      | TRUE=1
      |
      | Flags:
      | AMR_speed_measued = double() => Captura a velocidade do AMR
      | AMR_target_angle = double() => Captura o ângulo entre o AMR e o próximo waypoing
      | AMR_near_impact = TRUE => Sensor acusa impacto iminente
      | AMR_near_impact = FALSE => Sensor de impacto diz que está livre
      | AMR_ext_safety_plc = TRUE => Estado de emergência foi resolvido
      | AMR_ext_safety_plc = FALSE => Estado de emergência não foi resolvido
      | AMR_closedGate_ahead = TRUE => Existe um portão fechado a frente
      | AMR_closedGate_ahead = FALSE => Caminho livre
      | AMR_withLoad = TRUE => AMR está com carga (segue para estado de unloading)
      | AMR_withLoad = FALSE => AMR está sem carga (segue para o estado de loading)
      | AMR_inDestination = TRUE => AMR chegou ao destino de carga ou descarga
      | AMR_inDestination = FAIL => AMR chegou ao destino de carga ou descarga
      | AMR_system_startup = WAITING => AMR não foi inicializado (aguardando)
      | AMR_system_startup = SUCCESS => AMR inicializado com sucesso
      | AMR_system_startup = FAIL => AMR inicializado com falha
      | AMR_system_emergency = TRUE => AMR vai para modo de emergência
      | AMR_system_emergency = FALSE => AMR continua sua operação normal
      | AMR_manual_mode = TRUE => AMR vai para modo manual
      | AMR_manual_mode = FALSE => AMR continua sua operação normal
      | AMR_routeDefined = TRUE => AMR com rota definida
      | AMR_routeDefined = FALSE => AMR sem rota definida
  state S0_startup
    entry:
    state = 0;
    moving = 0;
    settings: description=This state models the modes of a window sensor and implements logic to respond when that sensor is producing a signal.
  state autonomousOperation
    settings: description=This state models the modes of a window sensor and implements logic to respond when that sensor is producing a signal.
    state S2_engaged
      entry:
      state = 2;
      settings: description=This state models the modes of a window sensor and implements logic to respond when that sensor is producing a signal.
      state S2A_Rotation
        entry:
        moving = 1;
      state S2B_Moving
        entry:
        moving = 2;
      state S2C_Parking
        entry:
        moving = 3;
      state S2D_Stopped
        entry:
        moving = 0;
      state S2E_Gate
        entry:
        moving = 0;
      (default) -> S2A_Rotation
      S2B_Moving -> (junction 285) [order 1] : [AMR_near_impact == TRUE]
      (junction 285) -> (junction 290)
      S2A_Rotation -> S2B_Moving : [AMR_target_angle <= 30]
      S2B_Moving -> S2C_Parking [order 2] : [AMR_target_angle > 30 | AMR_closedGate_ahead==TRUE | AMR_inDestination == TRUE]
      (junction 300) -> S2A_Rotation
      S2C_Parking -> (junction 290) [order 1] : [AMR_near_impact == TRUE]
      (junction 290) -> (junction 286)
      (junction 299) -> (junction 300)
      S2E_Gate -> (junction 300) [order 2] : [AMR_closedGate_ahead==TRUE]
      (junction 295) -> (junction 299) [order 3]
      S2C_Parking -> S2D_Stopped [order 2] : [AMR_measured_speed < 0.05]
      S2E_Gate -> S2E_Gate [order 1] : after(60, sec)
      (junction 295) -> S2E_Gate [order 2] : [AMR_closedGate_ahead==TRUE]
      S2D_Stopped -> (junction 295) : [AMR_near_impact == FALSE && AMR_measured_speed < 0.05]
      (junction 286) -> S2D_Stopped
    state S1_standby
      entry:
      state = 1;
      settings: description=This state models the modes of a window sensor and implements logic to respond when that sensor is producing a signal.
    state S4_unloading
      entry:
      state = 4;
      settings: description=This state models the modes of a window sensor and implements logic to respond when that sensor is producing a signal.
    state S3_loading
      entry:
      state = 3;
      settings: description=This state models the modes of a window sensor and implements logic to respond when that sensor is producing a signal.
    (default) -> S1_standby
    S1_standby -> S2_engaged : [AMR_routeDefined == TRUE]
    S4_unloading -> S1_standby
    (junction 269) -> S2_engaged
    S3_loading -> (junction 269)
    (junction 295) -> (junction 253) [order 1] : [AMR_inDestination==TRUE]
    (junction 275) -> S4_unloading
    (junction 254) -> S3_loading [order 1] : [AMR_withLoad == FALSE]
    (junction 254) -> (junction 275) [order 2] : [AMR_withLoad == TRUE]
    (junction 253) -> (junction 254)
  state E1_failed
    entry:
    state = -1;
    moving = 0;
    settings: description=This state models the modes of a window sensor and implements logic to respond when that sensor is producing a signal.
  state E2_emergency
    entry:
    state = -2;
    moving = 0;
    settings: description=This state models the modes of a window sensor and implements logic to respond when that sensor is producing a signal.
  state E3_manualMode
    entry:
    state = -3;
    moving = 0;
    settings: description=This state models the modes of a window sensor and implements logic to respond when that sensor is producing a signal.
  (default) -> (junction 244)
  (junction 242) -> (junction 244)
  (junction 244) -> S0_startup
  (junction 312) -> (junction 242)
  S0_startup -> (junction 257) : [AMR_system_start ~= WAITING]
  (junction 257) -> (junction 251) [order 1] : [AMR_system_start == FAIL]
  (junction 257) -> autonomousOperation [order 2] : [AMR_system_start == SUCCESS]
  (junction 251) -> E1_failed
  autonomousOperation -> E1_failed [order 3] : [AMR_system_start == FAIL]
  E1_failed -> (junction 312)
  (junction 243) -> (junction 312)
  E2_emergency -> (junction 243) [order 1] : [AMR_ext_safety_plc == TRUE]
  autonomousOperation -> E2_emergency [order 1] : [AMR_set_emergency == TRUE]
  E2_emergency -> E2_emergency [order 2] : after(10, sec)
  autonomousOperation -> E3_manualMode [order 2] : [AMR_manual_mode==TRUE | AMR_idle_mode==TRUE]
  E3_manualMode -> autonomousOperation : [AMR_manual_mode == FALSE]
  data: state output =0; moving output; FAIL constant double =-1; SUCCESS constant double =1; WAITING constant double =0; AMR_closedGate_ahead input; AMR_ext_safety_plc input; AMR_inDestination input; AMR_manual_mode input; AMR_idle_mode input; AMR_measured_speed input; AMR_near_impact input; AMR_set_emergency input; AMR_system_start input; AMR_target_angle input; AMR_withLoad input; FALSE constant double =0; TRUE constant double =1; AMR_routeDefined input
